simulink model "ButtonControlApp_Client"  (R2023a)
settings: Solver=FixedStepAuto  StartTime=0.0  StopTime=10.0  RelTol=1e-3
undefined symbols (not defined in the file): Data_Display1, ReceiveData
libraries: androidcommunicationlib x2, androiduilib x1
settings Model: Creator=aqeel  LastModifiedBy=aqeel
settings OptimizationCC: EnhancedBackFolding=on  PassReuseOutputArgsAs=Individual arguments  ZeroExternalMemoryAtStartup=off  ZeroInternalMemoryAtStartup=off  MaxStackSize=64  OptimizeBlockOrder=speed  DifferentSizesBufferReuse=on  OptimizationCustomize=off  EfficientTunableParamExpr=on
settings DebuggingCC: ParameterTunabilityLossMsg=error
settings HardwareCC: ProdBitPerPointer=32  ProdBitPerSizeT=32  ProdBitPerPtrDiffT=32  ProdLargestAtomicInteger=Long  ProdLargestAtomicFloat=Double  ProdWordSize=32  ProdHWDeviceType=ARM Compatible->ARM Cortex
settings SFSimCC: MATLABDynamicMemAlloc=off
settings RTWCC: Description=Embedded Coder  SystemTargetFile=ert.tlc  HardwareBoard=Android Device  TLCOptions="-aInlineSetEventsForThisBaseRateFcn=TLC_FALSE -aSuppressMultiTaskScheduler=TLC_FALSE  -aRateBasedStepFcn=0"  TemplateMakefile=ert_default_tmf  RTWVerbose=off  Toolchain=Android SDK/NDK Tools
settings CodeAppCC: ForceParamTrailComments=on  IgnoreCustomStorageClasses=off  OperatorAnnotations=on  SimulinkDataObjDesc=on  SFDataObjDesc=on  InsertBlockDesc=on

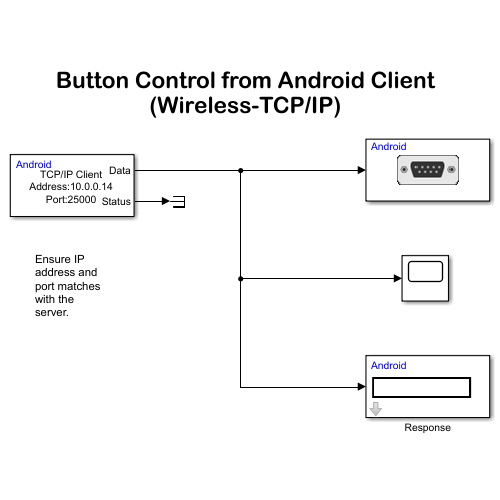
[thumbnail: Simulink's stored preview of the top-level diagram]
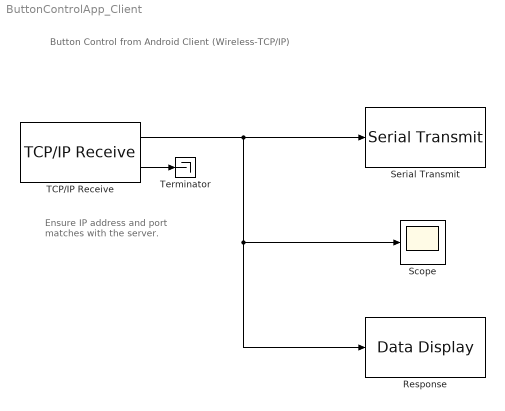
== system ButtonControlApp_Client ==
  note: Button Control from Android Client (Wireless-TCP/IP)
  note: Ensure IP address and port matches with the server.
  Response : androiduilib/Data Display  DataDisplayId=ReceiveData/Data_Display1  Format=Float  Precision=6  SimulateUsing=Code generation  blockPlatform=Android
  Scope : Scope
  Serial Transmit : androidcommunicationlib/Serial Transmit
  TCP/IP Receive : androidcommunicationlib/TCP//IP Receive  TCPReceiveId=ReceiveData/TCP//IP_Receive  Mode_=Client  LocalServerPort_=25000  RemoteAddr_=10.0.0.14  RemoteServerPort_=25000  DataType_=uint8  DataSize_=1  SampleTime_=0.1  ClientPortBindingSelection_=off  ClientPortToBind_=35000  BlockingMode_=off  BlockTimeout_=0.1
  Terminator : Terminator
  wires:
  TCP/IP Receive/1 -> Response/1, Scope/1, Serial Transmit/1
  TCP/IP Receive/2 -> Terminator/1
